simulink model "lab04"  (Simulink 7.4)
settings: Solver=ode45  StartTime=0.0  StopTime=10.0  RelTol=1e-3
libraries: cstblocks x16
settings Model: Creator=AshfaqAhmad  LastModifiedBy=AshfaqAhmad

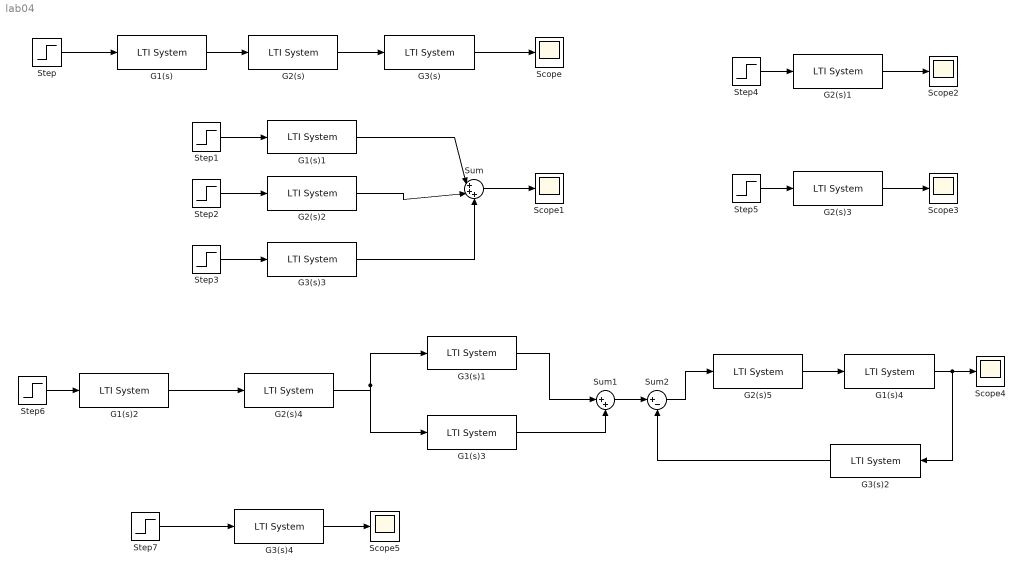
== system lab04 ==
  G1(s){,1..4} (5 alike) : cstblocks/LTI System  SystemSampleTime=-1  sys=tf(1,[1 1])  IC=[]
  G2(s){,2,4..5} (4 alike) : cstblocks/LTI System  SystemSampleTime=-1  sys=tf(1,[1 3])  IC=[]
  G2(s)1 : cstblocks/LTI System  SystemSampleTime=-1  sys=tf([1 3],[1 9 23 15])  IC=[]
  G2(s)3 : cstblocks/LTI System  SystemSampleTime=-1  sys=tf([1 9 29 29],[1 9 23 15])  IC=[]
  G3(s){,1..3} (4 alike) : cstblocks/LTI System  SystemSampleTime=-1  sys=tf([1 3],[1 5])  IC=[]
  G3(s)4 : cstblocks/LTI System  SystemSampleTime=-1  sys="tf([1 5],[1 13 63 141 144  54])"  IC=[]
  Scope{,1..5} (6 alike) : Scope
      Scope2 settings: SaveName=ScopeData2
      Scope3 settings: SaveName=ScopeData3
      Scope4 settings: SaveName=ScopeData4
      Scope5 settings: SaveName=ScopeData5
  Step{,1..7} (8 alike) : Step  SampleTime=0
  Sum : Sum  Inputs=|+++  OutDataType=fixdt(1, 16)  OutScaling=2^0
  Sum1 : Sum  Inputs=|++  OutDataType=fixdt(1, 16)  OutScaling=2^0
  Sum2 : Sum  Inputs=|+-  OutDataType=fixdt(1, 16)  OutScaling=2^0
  wires:
  G1(s)/1 -> G2(s)/1
  G2(s)/1 -> G3(s)/1
  Step/1 -> G1(s)/1
  G3(s)/1 -> Scope/1
  Step1/1 -> G1(s)1/1
  Step2/1 -> G2(s)2/1
  Step3/1 -> G3(s)3/1
  G1(s)1/1 -> Sum/1
  G2(s)2/1 -> Sum/2
  G3(s)3/1 -> Sum/3
  Sum/1 -> Scope1/1
  Step4/1 -> G2(s)1/1
  G2(s)1/1 -> Scope2/1
  Step5/1 -> G2(s)3/1
  G2(s)3/1 -> Scope3/1
  G1(s)2/1 -> G2(s)4/1
  G2(s)4/1 -> G3(s)1/1, G1(s)3/1
  G3(s)1/1 -> Sum1/1
  G1(s)3/1 -> Sum1/2
  Sum1/1 -> Sum2/1
  Sum2/1 -> G2(s)5/1
  G2(s)5/1 -> G1(s)4/1
  G1(s)4/1 -> Scope4/1, G3(s)2/1
  Step6/1 -> G1(s)2/1
  G3(s)2/1 -> Sum2/2
  Step7/1 -> G3(s)4/1
  G3(s)4/1 -> Scope5/1
